simulink model "ava3"  (R2017b)
settings: Solver=VariableStepAuto  StartTime=0.0  StopTime=10.0  RelTol=1e-3
model workspace (MAT data in the model file):
  const_EarthRate = 7.292115486e-05
  const_G_times_earth_mass = 398600441800000
  const_earth_equatorial_radius = 6378137
  const_earth_polar_radius = 6356752.3142
settings Model: Creator=hbourbou  LastModifiedBy=hbourbou

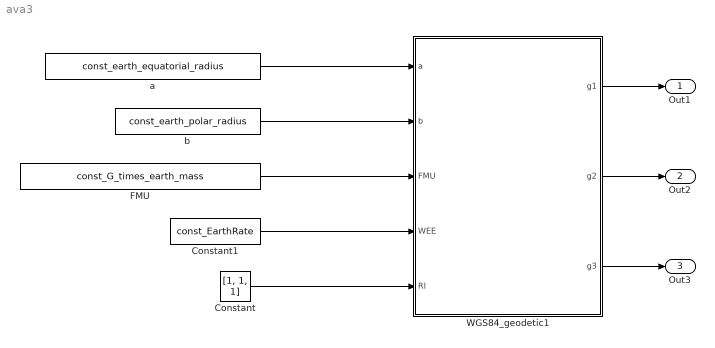
== system ava3 ==
  Constant : Constant  Value=[1, 1, 1]
  Constant1 : Constant  Value=const_EarthRate
  FMU : Constant  Value=const_G_times_earth_mass
  WGS84_geodetic1 : MATLAB Function  TreatAsAtomicUnit=on
  a : Constant  Value=const_earth_equatorial_radius
  b : Constant  Value=const_earth_polar_radius
  Out1 : Outport
  Out2 : Outport  Port=2
  Out3 : Outport  Port=3
  wires:
  a/1 -> WGS84_geodetic1/1(a)
  b/1 -> WGS84_geodetic1/2(b)
  FMU/1 -> WGS84_geodetic1/3(FMU)
  Constant/1 -> WGS84_geodetic1/5(RI)
  Constant1/1 -> WGS84_geodetic1/4(WEE)
  WGS84_geodetic1/1(g1) -> Out1/1
  WGS84_geodetic1/2(g2) -> Out2/1
  WGS84_geodetic1/3(g3) -> Out3/1

== matlab function ava3/WGS84_geodetic1 ==
  data: a input double; g1 output double; b input double; FMU input double; WEE input double; RI input double; g2 output double; g3 output double
%======================================================================C

function [g1,g2,g3] = wgs84(a, b, FMU, WEE, RI)
%#codegen
%(earth equatorial radius, polar radius, G*m_earth, earth rotation rate, inertial position vector)
%(output is acceleration)
%       SUBROUTINE WGS84 ( a, b, FMU, WEE, RI, g )
%======================================================================C
%                                                                      C
%  PURPOSE                                                             C
%  -------                                                             C
%  Computes the gravitational acceleration vector.  Model based on     C
%  algorithms defined in the following reference:                      C
%  "Department of Defense World Geodetic System, Its Definition and    C
%  Relationships with Local Geodetic Systems," National Imagery and    C
%  Mapping Agency (NIMA) Technical Report, TR8350.2, Third Addition,   C
%  Amendment 1, 3 January 2000. (Approved for Public Release)          C
%                                                                      C
%  INPUTS    DESCRIPTION                                               C
%                                                                      C
%   a        Earth semi-major axis (m)                                 C
%   b        Earth semi-minor axis (m)                                 C
%   FMU      Universal Gravitational Constant (m2/s3)                  C
%   WEE      Earth angular rate (rad/s)                                C
%   RI       Inertial position vector (m)                              C
%                                                                      C
%  OUTPUTS   DESCRIPTION                                               C
%                                                                      C
%    g       Gravitational acceleration vector (m/s2)                  C
%                                                                      C
%======================================================================C
%.....Define gravity model constants
%     Equation 4-7, pg. 4-3

      a2 = a*a;
      b2 = b*b;
      E2 = a2 - b2;
      E  = sqrt(E2);

%.....Equation 4-8, pg. 4-3
      x  = RI(1);
      y  = RI(2);
      z  = RI(3);
      x2 = x*x;
      y2 = y*y;
      z2 = z*z;
      u = 0.2;%sqrt(0.5*(x2 + y2 + z2 - E2)*(1.0 + sqrt(1.0 + 4.0*E2*z2/(x2 + y2 + z2 - E2)^2)));
      u2 = u*u;
      
%.....Equation 4-9, pg. 4-4
      beta = atan(z*sqrt(u2 + E2)/(u*sqrt(x2 + y2)));

%.....Equation 4-10, pg. 4-4
      SB = sin(beta);
      CB = cos(beta);
      w = sqrt((u2 + E2*SB*SB)/(u2 + E2));

%.....Equations 4-11 thru 4-13, pg. 4-4
      q  = 0.5*((1.0 + 3.0*u2/E2)*atan(E/u) - 3.0*u/E);
      q0 = 0.5*((1.0 + 3.0*b2/E2)*atan(E/b) - 3.0*b/E);
      qp = 3.0*(1.0 + u2/E2)*(1.0 - u/E*atan(E/u)) - 1.0;

%.....Equations 4-5 and 4-6, pg. 4-3
      omega = double(WEE);
      om2   = omega*omega;
      sque  = sqrt(u2 + E2);
      gamma_u = (-(FMU + om2*a2*E*qp*(0.5*SB*SB - 1.0/6.0)/q0)/(u2 + E2))/w;
      gamma_b = (a2*q/(q0*sque))*om2*SB*CB/w;
      gamma_l = 0.0;

%.....Rotate gravity to inertial frame - define rotation matrix,
%     equation 4-18, pg. 4-5
      xlam = atan2(y, x);
      clam = cos(xlam);
      slam = sin(xlam);
      R1=zeros(3,3);
      R1(1,1) =  u*CB*clam/(w*sque);
      R1(2,1) = -SB*clam/w;
      R1(3,1) = -slam;
      R1(1,2) =  u*CB*slam/(w*sque);
      R1(2,2) = -SB*slam/w;
      R1(3,2) =  clam;
      R1(1,3) =  SB/w;
      R1(2,3) =  u*CB/(w*sque);
      R1(3,3) =  0.0;
        
      %g=zeros(1,3);
      g1 = R1(1,1)*gamma_u + R1(2,1)*gamma_b + R1(3,1)*gamma_l;
      g2 = R1(1,2)*gamma_u + R1(2,2)*gamma_b + R1(3,2)*gamma_l;
      g3 = R1(1,3)*gamma_u + R1(2,3)*gamma_b + R1(3,3)*gamma_l;
      
end
